simulink model "MultirotorPX4Euler"  (R2020b)
settings: Solver=VariableStepAuto  StartTime=0.0  StopTime=100  RelTol=1e-3  EnableMultiTasking=on
PreLoadFcn:
  | InitializeParametersQuadcopterAIAAv3;
undefined symbols (not defined in the file or in its folder): Initial, Motor, Uav
settings Model: Creator=jban039  LastModifiedBy=jeremie
settings DataIOCC: Decimation=10
settings OptimizationCC: LifeSpan=inf
settings DebuggingCC: AllowSymbolicDim=off  SFUnexpectedBacktrackingDiag=warning  SFNoUnconditionalDefaultTransitionDiag=warning  SFExecutionAtInitializationDiag=none  ArithmeticOperatorsInVariantConditions=warning
settings ModelReferenceCC: ModelReferenceMinAlgLoopOccurrences=on  PropagateSignalLabelsOutOfModel=off
settings SFSimCC: SimUseLocalCustomCode=off  CustomCodeUndefinedFunction=UseInterfaceOnly
settings RTWCC: RTWUseLocalCustomCode=off
settings CodeAppCC: StateflowObjectComments=on
settings GRTTargetCC: TargetLangStandard=C89/C90 (ANSI)
settings ConfigComp: CovMetricSettings=dw  CovSaveCumulativeToWorkspaceVar=on  CovSaveSingleToWorkspaceVar=on  CovExternalEMLEnable=off

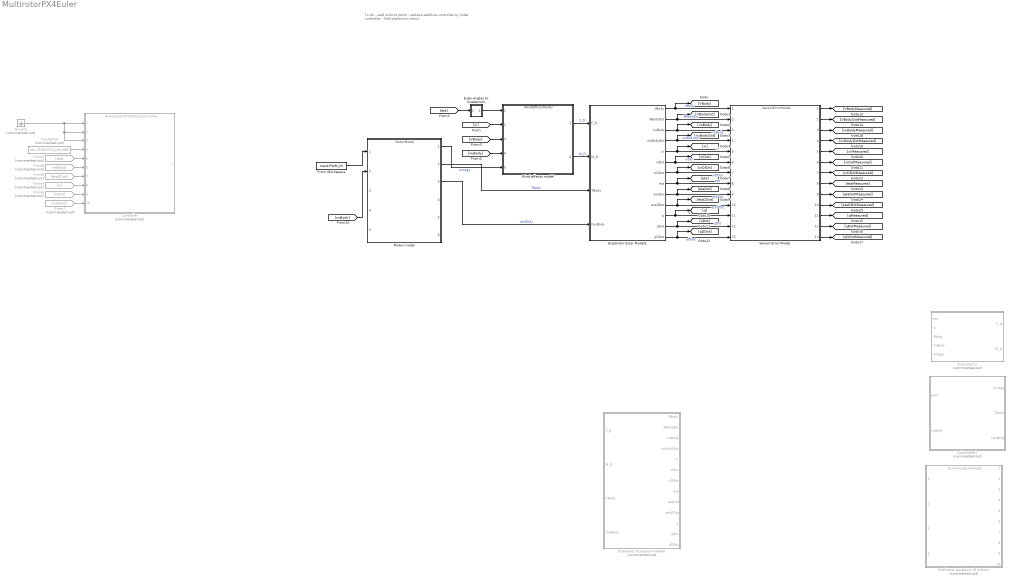
== system MultirotorPX4Euler ==
  note: To do:
      |
      | - add units  to ports
      | - replace stabilize controller by loiter controller
      | - Add quaternion eoms
  Constant4 : Constant  Commented=on  Value=Uav.THROTTLE_HOVER
  Controller : ModelReference  Commented=on  ModelNameDialog=ArduCopter33StabilizeController  SimulationMode=Normal  ModelReferenceVersion=1.9
  Euler Angles to Quaternion : Subsystem  AncestorBlock=QuaternionLibrary/Euler Angles to Quaternion
      mask help: Convert vector of Euler angles to an orientation quaternion
      mask Help:
      | Convert vector of Euler angles
      | [roll, pitch, yaw]
      | to an orientation quaternion
      | [q1 q2 q3 q4]
      | where:
      | - q1 is the rotation in radians
      | - [q2 q3 q4] is the vector around which the rotation is performed)
      | 
      | Based on code from the PX4 firmware: https://github.com/PX4/Firmware
      mask Display: disp('E2Q')
  From Workspace : FromWorkspace  VariableName=Input.PWM_IN
  From4 : From  Commented=on  GotoTag=xi
  From5 : From  Commented=on  GotoTag=eta
  From6 : From  Commented=on  GotoTag=xiDot
  From7 : From  Commented=on  GotoTag=xiDDot
  From8 : From  Commented=on  GotoTag=etaDot
  From9 : From  Commented=on  GotoTag=etaDDot
  Ground : Ground  Commented=on
  Motor model : ModelReference  ModelNameDialog=MotorModel  SimulationMode=Normal  ModelReferenceVersion=5.0
  Multirotor equations of motion : ModelReference  Commented=on  ModelNameDialog=QuadrotorEulerModel  SimulationMode=Normal  ModelReferenceVersion=5.0
  Quadrotor Euler Model1 : Subsystem
  Quadrotor Quaternion Model : Subsystem  Commented=on
  Sensor Error Model : ModelReference  ModelNameDialog=SensorErrorModel  SimulationMode=Normal  ModelReferenceVersion=5.0
  Subsystem1 : Subsystem  Commented=on
  Subsystem2 : Subsystem  Commented=on
  Wind effects model : ModelReference  ModelNameDialog=WindEffectsModel  SimulationMode=Normal  ModelReferenceVersion=1.55
  wires:
  Motor model/1 -> Wind effects model/5  "omega"
  Motor model/2 -> Quadrotor Euler Model1/3(TBody)  "TBody"
  Motor model/3 -> Quadrotor Euler Model1/4(tauBody)  "tauBody"
  Wind effects model/2 -> Quadrotor Euler Model1/2(M_D)  "M_D"
  Quadrotor Euler Model1/1(VBody) -> Sensor Error Model/1, [VBody]  "VBody"
  Quadrotor Euler Model1/2(VBodyDot) -> Sensor Error Model/2, [VBodyDot]  "VBodyDot"
  Quadrotor Euler Model1/3(nuBody) -> [nuBody], Sensor Error Model/3  "nuBody"
  Quadrotor Euler Model1/4(nuBodyDot) -> Sensor Error Model/4, [nuBodyDot]  "nuBodyDot"
  Quadrotor Euler Model1/5(xi) -> Sensor Error Model/5, [xi]  "xi"
  Quadrotor Euler Model1/6(xiDot) -> Sensor Error Model/6, [xiDot]  "xiDot"
  Quadrotor Euler Model1/7(xiDDot) -> Sensor Error Model/7, [xiDDot]  "xiDDot"
  Quadrotor Euler Model1/8(eta) -> Sensor Error Model/8, [eta]  "eta"
  Quadrotor Euler Model1/9(etaDot) -> Sensor Error Model/9, [etaDot]  "etaDot"
  Quadrotor Euler Model1/10(etaDDot) -> [etaDDot], Sensor Error Model/10  "etaDDot"
  [eta] -> Euler Angles to Quaternion/1(euler)
  [xi] -> Wind effects model/2
  [nuBody] -> Wind effects model/4
  [VBody] -> Wind effects model/3
  From5/1 -> Controller/5
  From4/1 -> Controller/8
  From6/1 -> Controller/9
  From7/1 -> Controller/10
  From8/1 -> Controller/6
  From9/1 -> Controller/7
  Ground/1 -> Controller/3, Controller/2, Controller/1
  Constant4/1 -> Controller/4
  [nuBody] -> Motor model/2
  From Workspace/1 -> Motor model/1
  Quadrotor Euler Model1/11(q) -> Sensor Error Model/11, [q]  "q"
  Quadrotor Euler Model1/12(qDot) -> [qDot], Sensor Error Model/12  "qDot"
  Quadrotor Euler Model1/13(qDDot) -> Sensor Error Model/13, [qDDot]  "qDDot"
  Wind effects model/1 -> Quadrotor Euler Model1/1(F_D)  "F_D"
  Sensor Error Model/1 -> [VBodyMeasured]
  Sensor Error Model/2 -> [VBodyDotMeasured]
  Sensor Error Model/3 -> [nuBodyMeasured]
  Sensor Error Model/4 -> [nuBodyDotMeasured]
  Sensor Error Model/5 -> [xiMeasured]
  Sensor Error Model/6 -> [xiDotMeasured]
  Sensor Error Model/7 -> [xiDDotMeasured]
  Sensor Error Model/8 -> [etaMeasured]
  Sensor Error Model/9 -> [etaDotMeasured]
  Sensor Error Model/10 -> [etaDDotMeasured]
  Sensor Error Model/11 -> [qMeasured]
  Sensor Error Model/12 -> [qDotMeasured]
  Sensor Error Model/13 -> [qDDotMeasured]
  Euler Angles to Quaternion/1(quaternion) -> Wind effects model/1

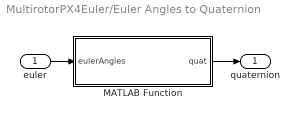
== system MultirotorPX4Euler/Euler Angles to Quaternion ==
  euler : Inport
  MATLAB Function : MATLAB Function  TreatAsAtomicUnit=on
  quaternion : Outport  VectorParamsAs1DForOutWhenUnconnected=off
  wires:
  MATLAB Function/1(quat) -> quaternion/1
  euler/1 -> MATLAB Function/1(eulerAngles)

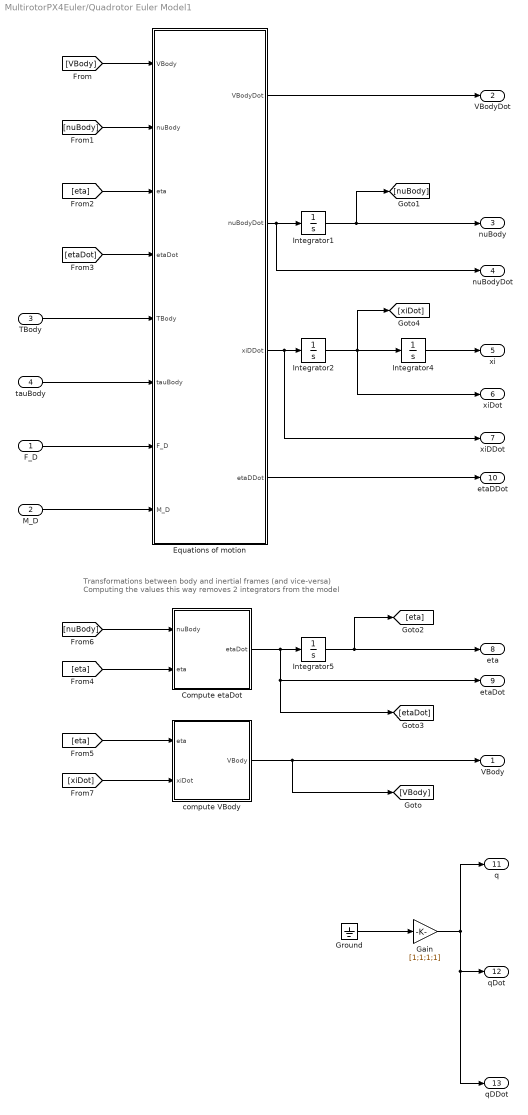
== system MultirotorPX4Euler/Quadrotor Euler Model1 ==
  note: Transformations between body and inertial frames (and vice-versa)
      | Computing the values this way removes 2 integrators from the model
  F_D : Inport
  M_D : Inport  Port=2
  TBody : Inport  Port=3
  tauBody : Inport  Port=4
  Compute etaDot : MATLAB Function  TreatAsAtomicUnit=on
  Equations of motion : MATLAB Function  TreatAsAtomicUnit=on
  Gain : Gain  Gain=[1;1;1;1]
  Ground : Ground
  Integrator1 : Integrator  InitialCondition=Initial.NU_BODY
  Integrator2 : Integrator  InitialCondition=Initial.XI_DOT
  Integrator4 : Integrator  InitialCondition=Initial.XI
  Integrator5 : Integrator  InitialCondition=Initial.ETA
  compute VBody : MATLAB Function  TreatAsAtomicUnit=on
  VBody : Outport  VectorParamsAs1DForOutWhenUnconnected=off
  VBodyDot : Outport  Port=2  VectorParamsAs1DForOutWhenUnconnected=off
  nuBody : Outport  Port=3  VectorParamsAs1DForOutWhenUnconnected=off
  nuBodyDot : Outport  Port=4  VectorParamsAs1DForOutWhenUnconnected=off
  xi : Outport  Port=5  VectorParamsAs1DForOutWhenUnconnected=off
  xiDot : Outport  Port=6  VectorParamsAs1DForOutWhenUnconnected=off
  xiDDot : Outport  Port=7  VectorParamsAs1DForOutWhenUnconnected=off
  eta : Outport  Port=8  VectorParamsAs1DForOutWhenUnconnected=off
  etaDot : Outport  Port=9  VectorParamsAs1DForOutWhenUnconnected=off
  etaDDot : Outport  Port=10  VectorParamsAs1DForOutWhenUnconnected=off
  q : Outport  Port=11  VectorParamsAs1DForOutWhenUnconnected=off
  qDot : Outport  Port=12  VectorParamsAs1DForOutWhenUnconnected=off
  qDDot : Outport  Port=13  VectorParamsAs1DForOutWhenUnconnected=off
  wires:
  [xiDot] -> compute VBody/2(xiDot)
  [nuBody] -> Compute etaDot/1(nuBody)
  Equations of motion/2(nuBodyDot) -> nuBodyDot/1, Integrator1/1
  Integrator1/1 -> nuBody/1, [nuBody]
  M_D/1 -> Equations of motion/8(M_D)
  [eta] -> compute VBody/1(eta)
  compute VBody/1(VBody) -> VBody/1, [VBody]
  [eta] -> Compute etaDot/2(eta)
  Compute etaDot/1(etaDot) -> etaDot/1, [etaDot], Integrator5/1
  F_D/1 -> Equations of motion/7(F_D)
  Equations of motion/4(etaDDot) -> etaDDot/1
  Equations of motion/3(xiDDot) -> xiDDot/1, Integrator2/1
  TBody/1 -> Equations of motion/5(TBody)
  tauBody/1 -> Equations of motion/6(tauBody)
  [etaDot] -> Equations of motion/4(etaDot)
  [eta] -> Equations of motion/3(eta)
  Integrator5/1 -> eta/1, [eta]
  [VBody] -> Equations of motion/1(VBody)
  [nuBody] -> Equations of motion/2(nuBody)
  Integrator4/1 -> xi/1
  Integrator2/1 -> xiDot/1, Integrator4/1, [xiDot]
  Equations of motion/1(VBodyDot) -> VBodyDot/1
  Ground/1 -> Gain/1
  Gain/1 -> q/1, qDDot/1, qDot/1

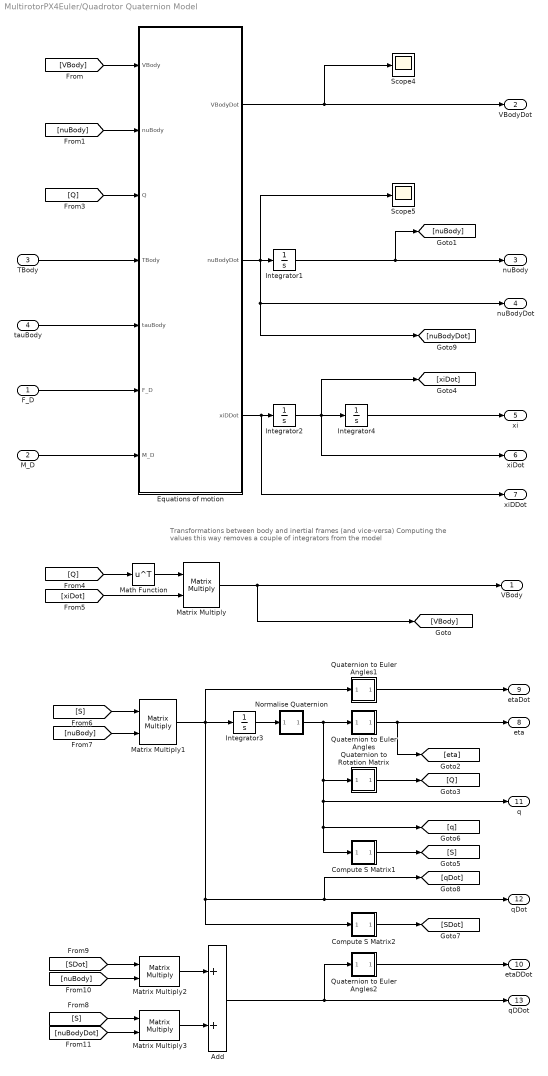
== system MultirotorPX4Euler/Quadrotor Quaternion Model ==
  note: Transformations between body and inertial frames (and vice-versa)
      | Computing the values this way removes a couple of integrators from the model
  F_D : Inport
  M_D : Inport  Port=2
  TBody : Inport  Port=3
  tauBody : Inport  Port=4
  Add : Sum
  Compute S Matrix1 : Subsystem  AncestorBlock=QuaternionLibrary/Compute S Matrix
      mask help: Convert an orientation quaternion to an orthogonal transformation matrix
      mask Help:
      | Convert a quaternion
      | [q1 q2 q3 q4]
      | to the S matrix used to compute angular acceleration and velocity quaternion
      | qDot = S * nuBody
      | 
      | qDDot = SDot * nuBody + S * nuBodyDot
      mask Display: disp('S')
  Compute S Matrix2 : Subsystem  AncestorBlock=QuaternionLibrary/Compute S Matrix
      mask help: Convert an orientation quaternion to an orthogonal transformation matrix
      mask Help:
      | Convert a quaternion
      | [q1 q2 q3 q4]
      | to the S matrix used to compute angular acceleration and velocity quaternion
      | qDot = S * nuBody
      | 
      | qDDot = SDot * nuBody + S * nuBodyDot
      mask Display: disp('S')
  Equations of motion : MATLAB Function  TreatAsAtomicUnit=on
  Integrator1 : Integrator  InitialCondition=Initial.NU_BODY
  Integrator2 : Integrator  InitialCondition=Initial.XI_DOT
  Integrator3 : Integrator  InitialCondition=[0;0;0;1]
  Integrator4 : Integrator  InitialCondition=Initial.XI
  Math Function : Math  Operator=transpose  SignedPower=on  SaturateOnIntegerOverflow=on
  Matrix Multiply{,1..3} (4 alike) : Product  Multiplication=Matrix(*)
  Normalise Quaternion : Subsystem  AncestorBlock=QuaternionLibrary/Normalise Quaternion
      mask help:
      | Normalise a quaternion
      |
      | Qhat = Q / |Q|
      mask Display: disp('Q/|Q|')
  Quaternion to Euler Angles : Subsystem  AncestorBlock=QuaternionLibrary/Quaternion to Euler Angles
      mask help: Convert an orientation quaternion to a vector of Euler angles
      mask Help:
      | Convert an orientation quaternion
      | [q1 q2 q3 q4]
      | where:
      | - q1 is the rotation in radians
      | - [q2 q3 q4] is the vector around which the rotation is performed)
      | to a vector of Euler angles
      | [roll, pitch, yaw]
      | Based on code from the PX4 firmware: https://github.com/PX4/Firmware
      mask Display: disp('Q2E')
  Quaternion to Euler Angles1 : Subsystem  AncestorBlock=QuaternionLibrary/Quaternion to Euler Angles
      mask help: Convert an orientation quaternion to a vector of Euler angles
      mask Help:
      | Convert an orientation quaternion
      | [q1 q2 q3 q4]
      | where:
      | - q1 is the rotation in radians
      | - [q2 q3 q4] is the vector around which the rotation is performed)
      | to a vector of Euler angles
      | [roll, pitch, yaw]
      | Based on code from the PX4 firmware: https://github.com/PX4/Firmware
      mask Display: disp('Q2E')
  Quaternion to Euler Angles2 : Subsystem  AncestorBlock=QuaternionLibrary/Quaternion to Euler Angles
      mask help: Convert an orientation quaternion to a vector of Euler angles
      mask Help:
      | Convert an orientation quaternion
      | [q1 q2 q3 q4]
      | where:
      | - q1 is the rotation in radians
      | - [q2 q3 q4] is the vector around which the rotation is performed)
      | to a vector of Euler angles
      | [roll, pitch, yaw]
      | Based on code from the PX4 firmware: https://github.com/PX4/Firmware
      mask Display: disp('Q2E')
  Quaternion to Rotation Matrix : Subsystem  AncestorBlock=QuaternionLibrary/Quaternion to Rotation Matrix
      mask help: Convert an orientation quaternion to an orthogonal transformation matrix
      mask Help:
      | Convert an orientation quaternion
      | [q1 q2 q3 q4]
      | where:
      | - q1 is the rotation in radians
      | - [q2 q3 q4] is the vector around which the rotation is performed)
      | to an orthogonal transformation matrix
      | Based on code from the PX4 firmware: https://github.com/PX4/Firmware
      mask Display: disp('Q2R')
  Scope4 : Scope
  Scope5 : Scope
  VBody : Outport  VectorParamsAs1DForOutWhenUnconnected=off
  VBodyDot : Outport  Port=2  VectorParamsAs1DForOutWhenUnconnected=off
  nuBody : Outport  Port=3  VectorParamsAs1DForOutWhenUnconnected=off
  nuBodyDot : Outport  Port=4  VectorParamsAs1DForOutWhenUnconnected=off
  xi : Outport  Port=5  VectorParamsAs1DForOutWhenUnconnected=off
  xiDot : Outport  Port=6  VectorParamsAs1DForOutWhenUnconnected=off
  xiDDot : Outport  Port=7  VectorParamsAs1DForOutWhenUnconnected=off
  eta : Outport  Port=8  VectorParamsAs1DForOutWhenUnconnected=off
  etaDot : Outport  Port=9  VectorParamsAs1DForOutWhenUnconnected=off
  etaDDot : Outport  Port=10  VectorParamsAs1DForOutWhenUnconnected=off
  q : Outport  Port=11  VectorParamsAs1DForOutWhenUnconnected=off
  qDot : Outport  Port=12  VectorParamsAs1DForOutWhenUnconnected=off
  qDDot : Outport  Port=13  VectorParamsAs1DForOutWhenUnconnected=off
  wires:
  Equations of motion/1(VBodyDot) -> VBodyDot/1, Scope4/1
  Integrator2/1 -> Integrator4/1, [xiDot], xiDot/1
  Integrator4/1 -> xi/1
  [nuBody] -> Equations of motion/2(nuBody)
  [VBody] -> Equations of motion/1(VBody)
  tauBody/1 -> Equations of motion/5(tauBody)
  TBody/1 -> Equations of motion/4(TBody)
  Equations of motion/3(xiDDot) -> Integrator2/1, xiDDot/1
  F_D/1 -> Equations of motion/6(F_D)
  Matrix Multiply/1 -> VBody/1, [VBody]
  M_D/1 -> Equations of motion/7(M_D)
  Integrator1/1 -> [nuBody], nuBody/1
  Equations of motion/2(nuBodyDot) -> Integrator1/1, nuBodyDot/1, [nuBodyDot], Scope5/1
  Integrator3/1 -> Normalise Quaternion/1(quaternion)
  Quaternion to Euler Angles/1(euler) -> eta/1, [eta]
  Quaternion to Euler Angles1/1(euler) -> etaDot/1
  Quaternion to Rotation Matrix/1(rotationMatrix) -> [Q]
  [Q] -> Equations of motion/3(Q)
  [Q] -> Math Function/1
  [xiDot] -> Matrix Multiply/2
  Math Function/1 -> Matrix Multiply/1
  [S] -> Matrix Multiply1/1
  [nuBody] -> Matrix Multiply1/2
  Compute S Matrix2/1(rotationMatrix) -> [SDot]
  [S] -> Matrix Multiply3/1
  Matrix Multiply1/1 -> Quaternion to Euler Angles1/1(quaternion), qDot/1, [qDot], Compute S Matrix2/1(quaternion), Integrator3/1
  [SDot] -> Matrix Multiply2/1
  [nuBody] -> Matrix Multiply2/2
  [nuBodyDot] -> Matrix Multiply3/2
  Matrix Multiply2/1 -> Add/1
  Matrix Multiply3/1 -> Add/2
  Add/1 -> Quaternion to Euler Angles2/1(quaternion), qDDot/1
  Normalise Quaternion/1(normalised) -> Quaternion to Euler Angles/1(quaternion), q/1, Compute S Matrix1/1(quaternion), [q], Quaternion to Rotation Matrix/1(quaternion)
  Compute S Matrix1/1(rotationMatrix) -> [S]
  Quaternion to Euler Angles2/1(euler) -> etaDDot/1

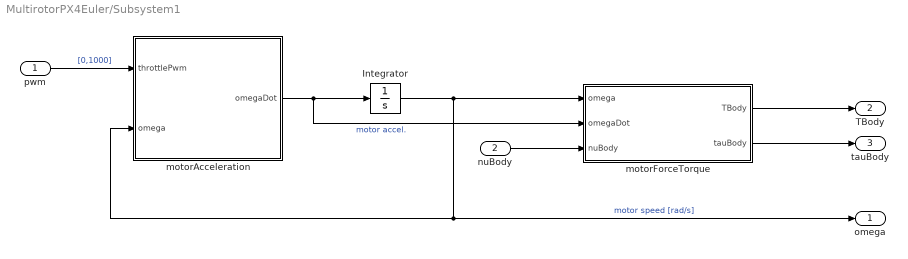
== system MultirotorPX4Euler/Subsystem1 ==
  pwm : Inport
  nuBody : Inport  Port=2
  Integrator : Integrator  InitialCondition=Initial.OMEGA
  motorAcceleration : MATLAB Function  TreatAsAtomicUnit=on
  motorForceTorque : MATLAB Function  TreatAsAtomicUnit=on
  omega : Outport  VectorParamsAs1DForOutWhenUnconnected=off
  TBody : Outport  Port=2  VectorParamsAs1DForOutWhenUnconnected=off
  tauBody : Outport  Port=3  VectorParamsAs1DForOutWhenUnconnected=off
  wires:
  motorAcceleration/1(omegaDot) -> motorForceTorque/2(omegaDot), Integrator/1  "motor accel."
  motorForceTorque/2(tauBody) -> tauBody/1
  motorForceTorque/1(TBody) -> TBody/1
  Integrator/1 -> motorForceTorque/1(omega), motorAcceleration/2(omega), omega/1  "motor speed [rad/s]"
  pwm/1 -> motorAcceleration/1(throttlePwm)  "[0,1000]"
  nuBody/1 -> motorForceTorque/3(nuBody)

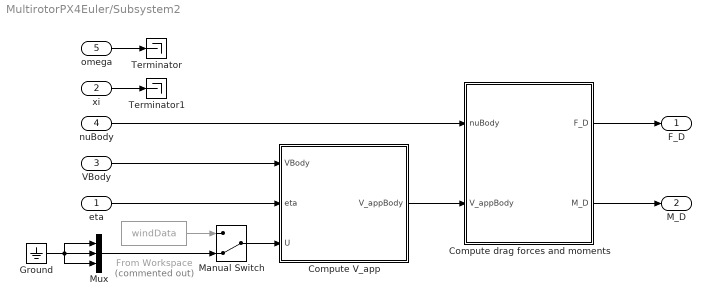
== system MultirotorPX4Euler/Subsystem2 ==
  eta : Inport  PortDimensions=3
  xi : Inport  Port=2  PortDimensions=3
  VBody : Inport  Port=3  PortDimensions=3
  nuBody : Inport  Port=4  PortDimensions=3
  omega : Inport  Port=5  PortDimensions=Uav.N_ROTORS
  Compute V_app : MATLAB Function  TreatAsAtomicUnit=on
  Compute drag forces and moments : MATLAB Function  TreatAsAtomicUnit=on
  From Workspace : FromWorkspace  Commented=on  VariableName=windData
  Ground : Ground
  Manual Switch : ManualSwitch  CurrentSetting=0
  Mux : Mux  Inputs=3
  Terminator : Terminator
  Terminator1 : Terminator
  F_D : Outport  VectorParamsAs1DForOutWhenUnconnected=off
  M_D : Outport  Port=2  VectorParamsAs1DForOutWhenUnconnected=off
  wires:
  Compute drag forces and moments/1(F_D) -> F_D/1
  Compute drag forces and moments/2(M_D) -> M_D/1
  Compute V_app/1(V_appBody) -> Compute drag forces and moments/2(V_appBody)
  omega/1 -> Terminator/1
  Manual Switch/1 -> Compute V_app/3(U)
  xi/1 -> Terminator1/1
  Ground/1 -> Mux/1, Mux/3, Mux/2
  From Workspace/1 -> Manual Switch/1
  Mux/1 -> Manual Switch/2
  nuBody/1 -> Compute drag forces and moments/1(nuBody)
  VBody/1 -> Compute V_app/1(VBody)
  eta/1 -> Compute V_app/2(eta)

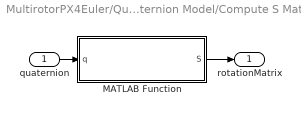
== system MultirotorPX4Euler/Quadrotor Quaternion Model/Compute S Matrix1 ==
  quaternion : Inport
  MATLAB Function : MATLAB Function  TreatAsAtomicUnit=on
  rotationMatrix : Outport  VectorParamsAs1DForOutWhenUnconnected=off
  wires:
  quaternion/1 -> MATLAB Function/1(q)
  MATLAB Function/1(S) -> rotationMatrix/1

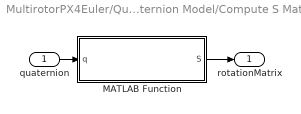
== system MultirotorPX4Euler/Quadrotor Quaternion Model/Compute S Matrix2 ==
  quaternion : Inport
  MATLAB Function : MATLAB Function  TreatAsAtomicUnit=on
  rotationMatrix : Outport  VectorParamsAs1DForOutWhenUnconnected=off
  wires:
  quaternion/1 -> MATLAB Function/1(q)
  MATLAB Function/1(S) -> rotationMatrix/1

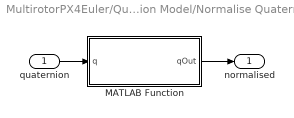
== system MultirotorPX4Euler/Quadrotor Quaternion Model/Normalise Quaternion ==
  quaternion : Inport
  MATLAB Function : MATLAB Function  TreatAsAtomicUnit=on
  normalised : Outport  VectorParamsAs1DForOutWhenUnconnected=off
  wires:
  quaternion/1 -> MATLAB Function/1(q)
  MATLAB Function/1(qOut) -> normalised/1

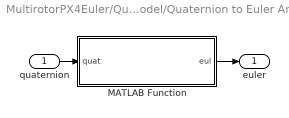
== system MultirotorPX4Euler/Quadrotor Quaternion Model/Quaternion to Euler Angles ==
  quaternion : Inport
  MATLAB Function : MATLAB Function  TreatAsAtomicUnit=on
  euler : Outport  VectorParamsAs1DForOutWhenUnconnected=off
  wires:
  quaternion/1 -> MATLAB Function/1(quat)
  MATLAB Function/1(eul) -> euler/1

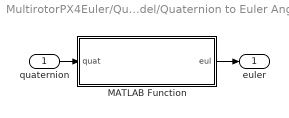
== system MultirotorPX4Euler/Quadrotor Quaternion Model/Quaternion to Euler Angles1 ==
  quaternion : Inport
  MATLAB Function : MATLAB Function  TreatAsAtomicUnit=on
  euler : Outport  VectorParamsAs1DForOutWhenUnconnected=off
  wires:
  quaternion/1 -> MATLAB Function/1(quat)
  MATLAB Function/1(eul) -> euler/1

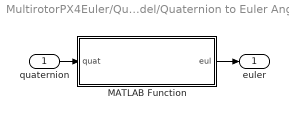
== system MultirotorPX4Euler/Quadrotor Quaternion Model/Quaternion to Euler Angles2 ==
  quaternion : Inport
  MATLAB Function : MATLAB Function  TreatAsAtomicUnit=on
  euler : Outport  VectorParamsAs1DForOutWhenUnconnected=off
  wires:
  quaternion/1 -> MATLAB Function/1(quat)
  MATLAB Function/1(eul) -> euler/1

== system MultirotorPX4Euler/Quadrotor Quaternion Model/Quaternion to Rotation Matrix ==
  quaternion : Inport
  MATLAB Function : MATLAB Function  TreatAsAtomicUnit=on
  rotationMatrix : Outport  VectorParamsAs1DForOutWhenUnconnected=off
  wires:
  MATLAB Function/1(R) -> rotationMatrix/1
  quaternion/1 -> MATLAB Function/1(q)

== matlab function MultirotorPX4Euler/Quadrotor Euler Model1/compute VBody ==
  data: eta input; VBody output; xiDot input
function VBody = computeVBody(eta, xiDot)
%#codegen

sphi = sin(eta(1));
sTheta = sin(eta(2));
sPsi = sin(eta(3));
cPhi = cos(eta(1));
cTheta = cos(eta(2));
cPsi = cos(eta(3));

R = [ cPsi*cTheta, cPsi*sTheta*sphi-sPsi*cPhi, cPsi*sTheta*cPhi+sPsi*sphi;
	  sPsi*cTheta, sPsi*sTheta*sphi+cPsi*cPhi, sPsi*sTheta*cPhi-cPsi*sphi;
     -sTheta,      cTheta*sphi,                cTheta*cPhi+sPsi*sphi];

VBody = R'*xiDot;

== matlab function MultirotorPX4Euler/Quadrotor Quaternion Model/Quaternion to Rotation Matrix/MATLAB Function ==
  data: q input; R output
function R = QuatToRot( q )
%QUATTOROT Convert quaternion to rotation matrix
%   Written by:    J.X.J. Bannwarth, 2017/03/27
%   Last modified: J.X.J. Bannwarth, 2018/12/11
    W = q(1);
    X = q(2);
    Y = q(3);
    Z = q(4);
    
    xx = X * X;
    xy = X * Y;
    xz = X * Z;
    xw = X * W;

    yy = Y * Y;
    yz = Y * Z;
    yw = Y * W;
    
    zz = Z * Z;
    zw = Z * W;

    m00 = 1 - 2 * ( yy + zz );
    m01 =     2 * ( xy - zw );
    m02 =     2 * ( xz + yw );

    m10 =     2 * ( xy + zw );
    m11 = 1 - 2 * ( xx + zz );
    m12 =     2 * ( yz - xw );

    m20 =     2 * ( xz - yw );
    m21 =     2 * ( yz + xw );
    m22 = 1 - 2 * ( xx + yy );
    
    R = [m00 m01 m02;
         m10 m11 m12;
         m20 m21 m22];   
end

== matlab function MultirotorPX4Euler/Euler Angles to Quaternion/MATLAB Function ==
  data: eulerAngles input; quat output
function quat   = EulerToQuaternion( eulerAngles )
%EULERTOQUATERNION Convert Euler angles to a quaternion
%   Based on PX4 Firmware code: https://github.com/PX4/Firmware
%   Written by: J.X.J. Bannwarth
%   Last modified: 29/08/2016

    roll  = eulerAngles(1);
    pitch = eulerAngles(2);
    yaw   = eulerAngles(3);

    cosPhi_2   = cos(roll / 2.0);
    sinPhi_2   = sin(roll / 2.0);
    cosTheta_2 = cos(pitch / 2.0);
    sinTheta_2 = sin(pitch / 2.0);
    cosPsi_2   = cos(yaw / 2.0);
    sinPsi_2   = sin(yaw / 2.0);

    quat = [ cosPhi_2 .* cosTheta_2 .* cosPsi_2 + sinPhi_2 .* sinTheta_2 .* sinPsi_2;
             sinPhi_2 .* cosTheta_2 .* cosPsi_2 - cosPhi_2 .* sinTheta_2 .* sinPsi_2;
             cosPhi_2 .* sinTheta_2 .* cosPsi_2 + sinPhi_2 .* cosTheta_2 .* sinPsi_2;
             cosPhi_2 .* cosTheta_2 .* sinPsi_2 - sinPhi_2 .* sinTheta_2 .* cosPsi_2 ];

end

== matlab function MultirotorPX4Euler/Quadrotor Quaternion Model/Quaternion to Euler Angles/MATLAB Function ==
  data: quat input; eul output
function eul   = QuaternionToEuler( quat )
%QUATERNIONTOEULER Convert quaternion to euler angles
%   Based on PX4 Firmware code: https://github.com/PX4/Firmware
%   Written by:    J.X.J. Bannwarth, 2016/08/29
%   Last modified: J.X.J. Bannwarth, 2018/12/11

    eul = [ atan2(2.0 .* (quat(1) .* quat(2) + quat(3) .* quat(4)), ...
                1.0 - 2.0 .* (quat(2) .* quat(2) + quat(3) .* quat(3)));
	        asin(2.0 .* (quat(1) .* quat(3) - quat(4) .* quat(2)));
            atan2(2.0 .* (quat(1) .* quat(4) + quat(2) .* quat(3)), ...
                1.0 - 2.0 .* (quat(3) .* quat(3) + quat(4) .* quat(4))) ];
end

== matlab function MultirotorPX4Euler/Quadrotor Quaternion Model/Quaternion to Euler Angles1/MATLAB Function ==
  data: quat input; eul output
function eul   = QuaternionToEuler( quat )
%QUATERNIONTOEULER Convert quaternion to euler angles
%   Based on PX4 Firmware code: https://github.com/PX4/Firmware
%   Written by:    J.X.J. Bannwarth, 2016/08/29
%   Last modified: J.X.J. Bannwarth, 2018/12/11

    eul = [ atan2(2.0 .* (quat(1) .* quat(2) + quat(3) .* quat(4)), ...
                1.0 - 2.0 .* (quat(2) .* quat(2) + quat(3) .* quat(3)));
	        asin(2.0 .* (quat(1) .* quat(3) - quat(4) .* quat(2)));
            atan2(2.0 .* (quat(1) .* quat(4) + quat(2) .* quat(3)), ...
                1.0 - 2.0 .* (quat(3) .* quat(3) + quat(4) .* quat(4))) ];
end

== matlab function MultirotorPX4Euler/Quadrotor Quaternion Model/Compute S Matrix1/MATLAB Function ==
  data: q input; S output
function S = ComputeSMatrix(q)
%COMPUTESMATRIX Compute S Matrix
%   Written by:    J.X.J. Bannwarth, 2017/03/28
%   Last modified: J.X.J. Bannwarth, 2018/12/11
    S = zeros( 4, 3 );
    S(1,1) = -q(2) * 0.5;
    S(1,2) = -q(3) * 0.5;
    S(1,3) = -q(4) * 0.5;
    S(2,1) =  q(1) * 0.5;
    S(2,2) = -q(4) * 0.5;
    S(2,3) =  q(3) * 0.5;
    S(3,1) =  q(4) * 0.5;
    S(3,2) =  q(1) * 0.5;
    S(3,3) = -q(2) * 0.5;
    S(4,1) = -q(3) * 0.5;
    S(4,2) =  q(2) * 0.5;
    S(4,3) =  q(1) * 0.5;
end

== matlab function MultirotorPX4Euler/Quadrotor Quaternion Model/Normalise Quaternion/MATLAB Function ==
  data: q input; qOut output
function qOut = NormaliseQuat( q )
%NORMALISEQUAT Normalise quaternion
%   Based on PX4 Firmware code: https://github.com/PX4/Firmware
%   Written by:    J.X.J. Bannwarth, 2018/12/11
%   Last modified: J.X.J. Bannwarth, 2018/12/11

    qOut = zeros(4,1);
    normVal = sqrt( dot( q, q ) );
    if normVal ~= 0
        qOut = q ./ normVal;
    end
end

== matlab function MultirotorPX4Euler/Quadrotor Quaternion Model/Compute S Matrix2/MATLAB Function ==
  data: q input; S output
function S = ComputeSMatrix(q)
%COMPUTESMATRIX Compute S Matrix
%   Written by:    J.X.J. Bannwarth, 2017/03/28
%   Last modified: J.X.J. Bannwarth, 2018/12/11
    S = zeros( 4, 3 );
    S(1,1) = -q(2) * 0.5;
    S(1,2) = -q(3) * 0.5;
    S(1,3) = -q(4) * 0.5;
    S(2,1) =  q(1) * 0.5;
    S(2,2) = -q(4) * 0.5;
    S(2,3) =  q(3) * 0.5;
    S(3,1) =  q(4) * 0.5;
    S(3,2) =  q(1) * 0.5;
    S(3,3) = -q(2) * 0.5;
    S(4,1) = -q(3) * 0.5;
    S(4,2) =  q(2) * 0.5;
    S(4,3) =  q(1) * 0.5;
end

== matlab function MultirotorPX4Euler/Quadrotor Quaternion Model/Quaternion to Euler Angles2/MATLAB Function ==
  data: quat input; eul output
function eul   = QuaternionToEuler( quat )
%QUATERNIONTOEULER Convert quaternion to euler angles
%   Based on PX4 Firmware code: https://github.com/PX4/Firmware
%   Written by:    J.X.J. Bannwarth, 2016/08/29
%   Last modified: J.X.J. Bannwarth, 2018/12/11

    eul = [ atan2(2.0 .* (quat(1) .* quat(2) + quat(3) .* quat(4)), ...
                1.0 - 2.0 .* (quat(2) .* quat(2) + quat(3) .* quat(3)));
	        asin(2.0 .* (quat(1) .* quat(3) - quat(4) .* quat(2)));
            atan2(2.0 .* (quat(1) .* quat(4) + quat(2) .* quat(3)), ...
                1.0 - 2.0 .* (quat(3) .* quat(3) + quat(4) .* quat(4))) ];
end

== matlab function MultirotorPX4Euler/Subsystem1/motorForceTorque ==
  data: omega input; TBody output; omegaDot input; nuBody input size=3; Motor parameter; Uav parameter; tauBody output
function [TBody, tauBody] = motorForceTorque(...
    omega, omegaDot, nuBody, Motor, Uav)
%#codegen

% Make assertions to avoid code generation errors
assert(Uav.N_ROTORS < 16);

%% Thrust and differential torque

% Concatenated motor force/torque vectors in respective motor frame
% eg. TMotor = [TMotor1, TMotor2, ..., TMotorN]
% where: - N is the number of rotors
%        - TMotorx (x ∈ [1,2,...,N]) is the thrust generated by motor x in
%          its own frame of reference
TMotorIndividual = [ zeros(2, Uav.N_ROTORS);
           Motor.K * (omega'.^2) ];
tauMotorIndividual = [ zeros(2, Uav.N_ROTORS);
             Uav.ROTOR_DIRECTION .* ...
                 ( Motor.B*(omega'.^2) + Motor.I_R(3,3)*omegaDot' ) ];

% Initialise matrices to store motor force/torque vectors in body frame
TBodyIndividual   = zeros(3, Uav.N_ROTORS);
tauBodyIndividual = zeros(3, Uav.N_ROTORS);

% Calculate forces and moments from each motor in the body frame
for i = 1:Uav.N_ROTORS
    l = Uav.L(i);
    beta = Uav.BETA(i);
    
 	RMotorToBody = [ 0,            0,            l*sin(beta);
                     0,            0,           -l*cos(beta);
                    -l*sin(beta),  l*cos(beta),  0 ];

	% Motor force/torque vectors in body frame - need rotation matrix for
	% canted rotors(!)
	TBodyIndividual(:,i) = TMotorIndividual(:,i);
	tauBodyIndividual(:,i) = tauMotorIndividual(:,i) + ...
        RMotorToBody * TMotorIndividual(:,i);
end

%% Gyroscopic moments

% Concatenated gyroscopic moments for each rotor
M_GBodyIndividual = zeros(3, Uav.N_ROTORS);

% Concatenated motor speeds in their respective frames
omegaMotor = [ zeros(2, Uav.N_ROTORS);
               Uav.ROTOR_DIRECTION .* omega' ];
           
% Angular momentum in motor frame
H_MMotorSeparate = Motor.I_R * omegaMotor;

% Gyroscopic moment vectors in body frame
for i = 1:Uav.N_ROTORS
	M_GBodyIndividual(:,i) = cross(nuBody, H_MMotorSeparate(:,i));
end

M_GBody = sum(M_GBodyIndividual, 2);

%% Total torque and moment

% Total force/torque in body frame
TBody = sum(TBodyIndividual, 2);
tauBody = sum(tauBodyIndividual, 2) + M_GBody;

end

== matlab function MultirotorPX4Euler/Subsystem1/motorAcceleration ==
  data: throttlePwm input; omegaDot output double size=4; omega input; Motor parameter; Uav parameter
function omegaDot = motorAcceleration(throttlePwm, omega, Motor, Uav)
%#codegen

voltage = throttlePwm * Uav.NOMINAL_BATTERY_VOLTAGE / 1000;

% Motor current ignoring inductance
current = (voltage - Motor.K_E*omega) / Motor.R;

netTorque = (Motor.K_T * current) - (Motor.B * omega.^2);

% Motor angular acceleration
omegaDot = netTorque / Motor.I_R(3,3);

== matlab function MultirotorPX4Euler/Quadrotor Quaternion Model/Equations of motion ==
  data: VBody input; VBodyDot output; nuBody input; Q input; TBody input size=3; tauBody input size=3; F_D input size=3; M_D input size=3; nuBodyDot output; Uav parameter; xiDDot output
function [VBodyDot, nuBodyDot, xiDDot] = QuadrotorEulerModel(...
    VBody, nuBody, Q, TBody, tauBody, F_D, M_D, Uav)
%#codegen

%% Rotation matrices

%% Moments and Forces
% Body frame accelerations
VBodyDot  = (1/Uav.M) * (Q'*Uav.G + TBody - cross(nuBody, Uav.M*VBody) - F_D);
nuBodyDot = Uav.I \ (tauBody - cross(nuBody, Uav.I*nuBody) - M_D);

% Inertial frame accelerations
xiDDot = (1/Uav.M)*(Uav.G + Q*TBody - Q*F_D);
% etaDDot = WInvertDot*nuBody + WInvert*nuBodyDot;

% Check centripetal force in inertial frame
% F_C = R*cross(nuBody,m*VBody);
end

== matlab function MultirotorPX4Euler/Subsystem2/Compute V_app ==
  data: VBody input; eta input; V_appBody output; U input size=3
function V_appBody = computeV_appBody(VBody, eta, U)
%#codegen

sPhi   = sin(eta(1));
sTheta = sin(eta(2));
sPsi   = sin(eta(3));
cPhi   = cos(eta(1));
cTheta = cos(eta(2));
cPsi   = cos(eta(3));

R = [cPsi*cTheta, cPsi*sTheta*sPhi-sPsi*cPhi, cPsi*sTheta*cPhi+sPsi*sPhi;
     sPsi*cTheta, sPsi*sTheta*sPhi+cPsi*cPhi, sPsi*sTheta*cPhi-cPsi*sPhi;
     -sTheta,     cTheta*sPhi,                cTheta*cPhi+sPsi*sPhi];

% Rotation matrix from Wind frame to Inertial frame 
R_U = [1, 0,  0;
       0, 1,  0;
       0, 0, -1];

V_appBody = VBody + R'*R_U*U;

== matlab function MultirotorPX4Euler/Subsystem2/Compute drag forces and moments ==
  data: nuBody input; V_appBody input; F_D output; M_D output; Uav parameter
function [F_D, M_D] = computeDrag(nuBody, V_appBody, Uav)
%#codegen

% Calculate drag force
F_D = 0.5 * Uav.RHO_AIR * Uav.C_D * (abs(V_appBody) .* V_appBody);

% Drag moment, applied to independent axes
M_D = 0.5 * Uav.RHO_AIR * Uav.C_DM * (abs(nuBody) .* nuBody);

== matlab function MultirotorPX4Euler/Quadrotor Euler Model1/Compute etaDot ==
  data: nuBody input; eta input; etaDot output
function etaDot = computeEtaDot(nuBody, eta)
%#codegen

sPhi = sin(eta(1));
cPhi = cos(eta(1));
cTheta = cos(eta(2));
tTheta = tan(eta(2));
      
WInverse = [1, sPhi*tTheta,  cPhi*tTheta;
            0, cPhi,        -sPhi;
            0, sPhi/cTheta,  cPhi/cTheta];

etaDot = WInverse*nuBody;

== matlab function MultirotorPX4Euler/Quadrotor Euler Model1/Equations of motion ==
  data: VBody input; VBodyDot output; nuBody input; eta input; etaDot input; TBody input size=3; tauBody input size=3; F_D input size=3; M_D input size=3; nuBodyDot output; Uav parameter; xiDDot output; etaDDot output
function [VBodyDot, nuBodyDot, xiDDot, etaDDot] = QuadrotorEulerModel(...
    VBody, nuBody, eta, etaDot, TBody, tauBody, F_D, M_D, Uav)
%#codegen

%% Rotation matrices
% Precompute sines and cosines
sPhi   = sin(eta(1));
sTheta = sin(eta(2));
sPsi   = sin(eta(3));
cPhi   = cos(eta(1));
cTheta = cos(eta(2));
cPsi   = cos(eta(3));
tTheta = tan(eta(2));

phiDot   = etaDot(1);
thetaDot = etaDot(2);

% Body frame to inertial frame
R = [cPsi*cTheta, cPsi*sTheta*sPhi-sPsi*cPhi, cPsi*sTheta*cPhi+sPsi*sPhi;
     sPsi*cTheta, sPsi*sTheta*sPhi+cPsi*cPhi, sPsi*sTheta*cPhi-cPsi*sPhi;
     -sTheta,     cTheta*sPhi,                cTheta*cPhi+sPsi*sPhi];

WInvertDot = [...
    0,  phiDot*cPhi*tTheta+thetaDot*sPhi/cTheta^2,    -phiDot*sPhi*cTheta+thetaDot*cPhi/cTheta^2;
    0, -phiDot*sPhi,                                  -phiDot*cPhi;
	0,  phiDot*cPhi/cTheta+phiDot*sPhi*tTheta/cTheta, -phiDot*sPhi/cTheta+thetaDot*cPhi*tTheta/cTheta];

WInvert = [1, sPhi*tTheta,  cPhi*tTheta;
           0, cPhi,        -sPhi;
           0, sPhi/cTheta,  cPhi/cTheta];

%% Moments and Forces
% Body frame accelerations
VBodyDot  = (1/Uav.M) * (R'*Uav.G + TBody - cross(nuBody, Uav.M*VBody) - F_D);
nuBodyDot = Uav.I \ (tauBody - cross(nuBody, Uav.I*nuBody) - M_D);

% Inertial frame accelerations
xiDDot = (1/Uav.M)*(Uav.G + R*TBody - R*F_D);
etaDDot = WInvertDot*nuBody + WInvert*nuBodyDot;

% Check centripetal force in inertial frame
% F_C = R*cross(nuBody,m*VBody);
end

function S = computeS(q)
    S = 0.5 .* [-q(1), -q(2), -q(3);
                 q(0), -q(3),  q(2);
                 q(3),  q(0), -q(1);
                -q(2),  q(1),  q(0)];
end
